simulink model "Part1"  (R2024a)
settings: Solver=ode23t  StartTime=0.0  StopTime=1  RelTol=1e-3  AbsTol=1e-3
settings Model: Creator=apeer  LastModifiedBy=apeer
settings SolverCC: AutoScaleAbsTol=off  AlgebraicLoopSolver=TrustRegion  MaxZcPerStep=1
settings DebuggingCC: UnconnectedInputMsg=warning  UnconnectedOutputMsg=warning  UnconnectedLineMsg=warning  SymbolicDimsDataTypeCodeGenerationDiagnostic=none
settings ModelReferenceCC: EnableRefExpFcnMdlSchedulingChecks=on
settings SFSimCC: CustomCodeUndefinedFunction=UseInterfaceOnly
settings RTWCC: GPUComputeCapability=3.5  DLArmComputeVersion=19.05
settings SimscapeCC: SimscapeLogType=all  SimscapeLogSimulationStatistics=on  SimscapeLogDataHistory=10000

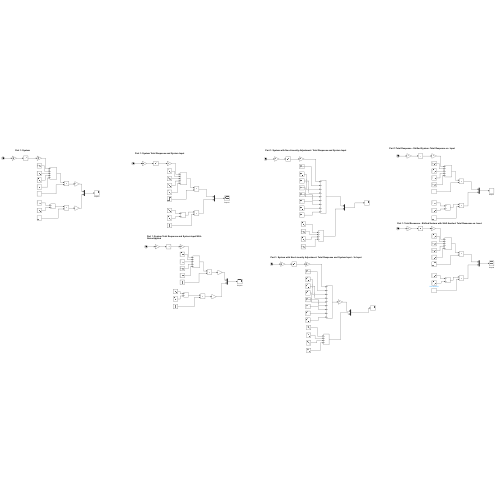
[thumbnail: Simulink's stored preview of the top-level diagram]
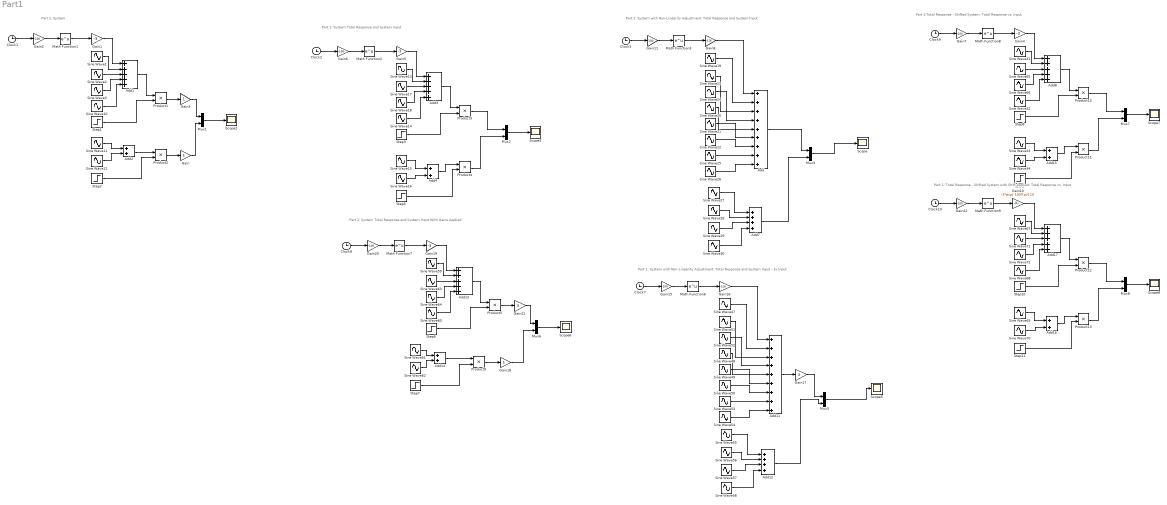
== system Part1 ==
  note: Part 1: System
  note: Part 1: System Total Response and System Input
  note: Part 1: System with Non-Linearity Adjustment: Total Response and System Input
  note: Part 1: System Total Response and System Input With Gains Applied
  note: Part 1: System with Non-Linearity Adjustment: Total Response and System Input - 3x Input
  note: Part 1:Total Response - Shifted System: Total Response vs. Input
  note: Part 1: Total Response - Shifted System with Shift Applied: Total Response vs. Input
  Add : Sum  Inputs=+++++++++
  Add{1,3,8,13,17} (5 alike) : Sum  Inputs=+++++
  Add11 : Sum  Inputs=+++++++++
  Add12 : Sum  Inputs=++++
  Add{2,4,14..16} (5 alike) : Sum
  Add7 : Sum  Inputs=++++
  Clock{1..2,5,7..10} (7 alike) : Clock
  Gain : Gain
  Gain{1,4..5,19} (4 alike) : Gain  Gain=-3
  Gain10 : Gain  Gain=-3*exp(-100*(pi/12))
  Gain{2,6..7,11,15,20,22} (7 alike) : Gain  Gain=-100
  Gain16 : Gain  Gain=-5.28
  Gain17 : Gain  Gain=3
  Gain18 : Gain
  Gain21 : Gain  Gain=3
  Gain3 : Gain
  Gain8 : Gain  Gain=-5.28
  Math Function{1..3,6..9} (7 alike) : Math
  Mux{1..3,5..8} (7 alike) : Mux  Inputs=2
  Product{1..5,9..13} (10 alike) : Product
  Scope{,2..3,5..8} (7 alike) : Scope
  Sine Wave1 : Sin  Amplitude=100/101  Frequency=10  Phase=pi/2  SampleTime=0
  Sine Wave10 : Sin  Amplitude=10/101  Frequency=1000  SampleTime=0
  Sine Wave11 : Sin  Frequency=10  Phase=pi/2  SampleTime=0
  Sine Wave12 : Sin  Frequency=1000  Phase=pi/2  SampleTime=0
  Sine Wave13 : Sin  Amplitude=100/101  Frequency=10  Phase=pi/2  SampleTime=0
  Sine Wave14 : Sin  Amplitude=10/101  Frequency=1000  SampleTime=0
  Sine Wave15 : Sin  Frequency=10  Phase=pi/2  SampleTime=0
  Sine Wave16 : Sin  Frequency=1000  Phase=pi/2  SampleTime=0
  Sine Wave17 : Sin  Amplitude=1/101  Frequency=1000  Phase=pi/2  SampleTime=0
  Sine Wave18 : Sin  Amplitude=10/101  Frequency=10  SampleTime=0
  Sine Wave19 : Sin  Amplitude=0.5  Frequency=20  Phase=pi/2  SampleTime=0
  Sine Wave2 : Sin  Amplitude=1/101  Frequency=1000  Phase=pi/2  SampleTime=0
  Sine Wave20 : Sin  Amplitude=0.025  Frequency=2000  SampleTime=0
  Sine Wave21 : Sin  Amplitude=0.01  Frequency=990  Phase=pi/2  SampleTime=0
  Sine Wave22 : Sin  Amplitude=0.1  Frequency=990  SampleTime=0
  Sine Wave23 : Sin  Amplitude=0.1  Frequency=20  SampleTime=0
  Sine Wave24 : Sin  Amplitude=1.26  Frequency=2000  Phase=pi/2  SampleTime=0
  Sine Wave25 : Sin  Amplitude=0.01  Frequency=1010  Phase=pi/2  SampleTime=0
  Sine Wave26 : Sin  Amplitude=0.1  Frequency=1010  SampleTime=0
  Sine Wave27 : Sin  Amplitude=1/2  Bias=1/2  Frequency=20  Phase=pi/2  SampleTime=0
  Sine Wave28 : Sin  Amplitude=1/2  Bias=1/2  Frequency=2000  Phase=pi/2  SampleTime=0
  Sine Wave29 : Sin  Frequency=990  Phase=pi/2  SampleTime=0
  Sine Wave3 : Sin  Amplitude=10/101  Frequency=10  SampleTime=0
  Sine Wave30 : Sin  Frequency=1010  Phase=pi/2  SampleTime=0
  Sine Wave31 : Sin  Amplitude=100/(20*sqrt(26))  Frequency=20  Phase=pi/2  SampleTime=0
  Sine Wave32 : Sin  Amplitude=100/2002.5  Frequency=2000  SampleTime=0
  Sine Wave33 : Sin  Frequency=20  Phase=pi/2  SampleTime=0
  Sine Wave34 : Sin  Frequency=2000  Phase=pi/2  SampleTime=0
  Sine Wave47 : Sin  Amplitude=0.5  Frequency=20  Phase=pi/2  SampleTime=0
  Sine Wave48 : Sin  Amplitude=0.025  Frequency=2000  SampleTime=0
  Sine Wave49 : Sin  Amplitude=0.01  Frequency=990  Phase=pi/2  SampleTime=0
  Sine Wave50 : Sin  Amplitude=0.1  Frequency=990  SampleTime=0
  Sine Wave51 : Sin  Amplitude=0.1  Frequency=20  SampleTime=0
  Sine Wave52 : Sin  Amplitude=1.26  Frequency=2000  Phase=pi/2  SampleTime=0
  Sine Wave53 : Sin  Amplitude=0.01  Frequency=1010  Phase=pi/2  SampleTime=0
  Sine Wave54 : Sin  Amplitude=0.1  Frequency=1010  SampleTime=0
  Sine Wave55 : Sin  Amplitude=9/2  Bias=9/2  Frequency=20  Phase=pi/2  SampleTime=0
  Sine Wave56 : Sin  Amplitude=9/2  Bias=9/2  Frequency=2000  Phase=pi/2  SampleTime=0
  Sine Wave57 : Sin  Amplitude=9  Frequency=990  Phase=pi/2  SampleTime=0
  Sine Wave58 : Sin  Amplitude=9  Frequency=1010  Phase=pi/2  SampleTime=0
  Sine Wave59 : Sin  Amplitude=100/101  Frequency=10  Phase=pi/2  SampleTime=0
  Sine Wave60 : Sin  Amplitude=10/101  Frequency=1000  SampleTime=0
  Sine Wave61 : Sin  Amplitude=3  Frequency=10  Phase=pi/2  SampleTime=0
  Sine Wave62 : Sin  Amplitude=3  Frequency=1000  Phase=pi/2  SampleTime=0
  Sine Wave63 : Sin  Amplitude=1/101  Frequency=1000  Phase=pi/2  SampleTime=0
  Sine Wave64 : Sin  Amplitude=10/101  Frequency=10  SampleTime=0
  Sine Wave65 : Sin  Amplitude=0.198  Frequency=20  SampleTime=0
  Sine Wave66 : Sin  Amplitude=2/801  Frequency=2000  Phase=pi/2  SampleTime=0
  Sine Wave67 : Sin  Amplitude=100/(20*sqrt(26))  Frequency=20  Phase=pi/2+(3*pi/12)  SampleTime=0
  Sine Wave68 : Sin  Amplitude=100/2002.5  Frequency=2000  Phase=+(3*pi/12)  SampleTime=0
  Sine Wave69 : Sin  Frequency=20  Phase=pi/2+(3*pi/12)  SampleTime=0
  Sine Wave70 : Sin  Frequency=2000  Phase=pi/2+(3*pi/12)  SampleTime=0
  Sine Wave71 : Sin  Amplitude=0.198  Frequency=20  Phase=+(3*pi/12)  SampleTime=0
  Sine Wave72 : Sin  Amplitude=2/801  Frequency=2000  Phase=pi/2+(3*pi/12)  SampleTime=0
  Step{1..3,5..11} (10 alike) : Step  Time=0  SampleTime=0
  wires:
  Step1/1 -> Product1/2
  Sine Wave10/1 -> Add1/5
  Add1/1 -> Product1/1
  Gain1/1 -> Add1/1
  Sine Wave3/1 -> Add1/4
  Gain2/1 -> Math Function1/1
  Math Function1/1 -> Gain1/1
  Clock1/1 -> Gain2/1
  Mux1/1 -> Scope2/1
  Sine Wave1/1 -> Add1/2
  Sine Wave2/1 -> Add1/3
  Add2/1 -> Product2/1
  Sine Wave12/1 -> Add2/2
  Step2/1 -> Product2/2
  Sine Wave11/1 -> Add2/1
  Gain/1 -> Mux1/2
  Product2/1 -> Gain/1
  Product1/1 -> Gain3/1
  Gain3/1 -> Mux1/1
  Sine Wave15/1 -> Add4/1
  Step5/1 -> Product4/2
  Sine Wave16/1 -> Add4/2
  Sine Wave17/1 -> Add3/3
  Sine Wave13/1 -> Add3/2
  Mux2/1 -> Scope3/1
  Sine Wave14/1 -> Add3/5
  Gain5/1 -> Add3/1
  Math Function2/1 -> Gain5/1
  Clock2/1 -> Gain6/1
  Sine Wave18/1 -> Add3/4
  Add3/1 -> Product3/1
  Step3/1 -> Product3/2
  Gain6/1 -> Math Function2/1
  Add4/1 -> Product4/1
  Clock5/1 -> Gain11/1
  Gain11/1 -> Math Function3/1
  Math Function3/1 -> Gain8/1
  Gain8/1 -> Add/1
  Sine Wave19/1 -> Add/2
  Sine Wave23/1 -> Add/3
  Sine Wave24/1 -> Add/4
  Sine Wave20/1 -> Add/5
  Sine Wave21/1 -> Add/6
  Sine Wave22/1 -> Add/7
  Sine Wave25/1 -> Add/8
  Sine Wave26/1 -> Add/9
  Sine Wave27/1 -> Add7/1
  Sine Wave28/1 -> Add7/2
  Sine Wave29/1 -> Add7/3
  Sine Wave30/1 -> Add7/4
  Mux3/1 -> Scope/1
  Add/1 -> Mux3/1
  Add7/1 -> Mux3/2
  Sine Wave47/1 -> Add11/2
  Sine Wave54/1 -> Add11/9
  Gain16/1 -> Add11/1
  Sine Wave51/1 -> Add11/3
  Math Function6/1 -> Gain16/1
  Sine Wave53/1 -> Add11/8
  Sine Wave49/1 -> Add11/6
  Gain15/1 -> Math Function6/1
  Clock7/1 -> Gain15/1
  Sine Wave48/1 -> Add11/5
  Add11/1 -> Gain17/1
  Sine Wave50/1 -> Add11/7
  Mux5/1 -> Scope5/1
  Sine Wave52/1 -> Add11/4
  Sine Wave55/1 -> Add12/1
  Sine Wave58/1 -> Add12/4
  Sine Wave56/1 -> Add12/2
  Sine Wave57/1 -> Add12/3
  Add12/1 -> Mux5/2
  Gain17/1 -> Mux5/1
  Step7/1 -> Product9/2
  Sine Wave62/1 -> Add14/2
  Gain18/1 -> Mux6/2
  Product9/1 -> Gain18/1
  Add14/1 -> Product9/1
  Add13/1 -> Product5/1
  Gain19/1 -> Add13/1
  Gain21/1 -> Mux6/1
  Clock8/1 -> Gain20/1
  Math Function7/1 -> Gain19/1
  Sine Wave61/1 -> Add14/1
  Mux6/1 -> Scope6/1
  Step6/1 -> Product5/2
  Sine Wave60/1 -> Add13/5
  Sine Wave59/1 -> Add13/2
  Sine Wave64/1 -> Add13/4
  Sine Wave63/1 -> Add13/3
  Gain20/1 -> Math Function7/1
  Product5/1 -> Gain21/1
  Product3/1 -> Mux2/1
  Product4/1 -> Mux2/2
  Product11/1 -> Mux7/2
  Step9/1 -> Product11/2
  Sine Wave34/1 -> Add15/2
  Add15/1 -> Product11/1
  Add8/1 -> Product10/1
  Gain4/1 -> Add8/1
  Clock9/1 -> Gain7/1
  Math Function8/1 -> Gain4/1
  Sine Wave33/1 -> Add15/1
  Sine Wave31/1 -> Add8/2
  Sine Wave66/1 -> Add8/4
  Sine Wave65/1 -> Add8/3
  Gain7/1 -> Math Function8/1
  Product10/1 -> Mux7/1
  Mux7/1 -> Scope7/1
  Step8/1 -> Product10/2
  Sine Wave32/1 -> Add8/5
  Sine Wave68/1 -> Add17/5
  Product12/1 -> Mux8/1
  Mux8/1 -> Scope8/1
  Step10/1 -> Product12/2
  Clock10/1 -> Gain22/1
  Sine Wave70/1 -> Add16/2
  Sine Wave69/1 -> Add16/1
  Gain22/1 -> Math Function9/1
  Math Function9/1 -> Gain10/1
  Add17/1 -> Product12/1
  Gain10/1 -> Add17/1
  Sine Wave71/1 -> Add17/3
  Sine Wave72/1 -> Add17/4
  Sine Wave67/1 -> Add17/2
  Step11/1 -> Product13/2
  Product13/1 -> Mux8/2
  Add16/1 -> Product13/1
